simulink model "M2C_IM_CL_V1_NCADMM_Sim"  (R2023a)
settings: Solver=ode4  StartTime=0.0  StopTime=t_sim  FixedStep=tsim  RelTol=1e-3
model workspace (MAT data in the model file):
  global_can_baud_rate = '1000000'
  global_ip_addresses : object (value not decoded)
values from neighbouring files (symbols this model uses):
  A = [1 1 1 0 0 0 ... (first row only)    [M2C_init.m]    (also in MMCC_Sim_Script_BCD_activeset.m = -[1 0 0 1 0 0 1 0 0; 0 1 0 0 1 0 0 1 0; 0 0 1 0 0 1 0 0 1; -; MMCC_Sim_Script_BCD_activeset_LH.m = -[1 0 0 1 0 0 1 0 0; 0 1 0 0 1 0 0 1 0; 0 0 1 0 0 1 0 0 1; -)
  A11 = -(1/tau_sig)*eye(2)    [M2C_init.m]
  A21 = (Lm/tau_r)*eye(2)    [M2C_init.m]
  A_admm = zeros(2*Np, Np)    [M2C_init.m]
  A_cc = [1 0 ... (first row only)    [M2C_init.m]
  b_admm_1 = imax_admm*ones(2*Np,1)    [M2C_init.m]
  b_cc = Vmax_cc*ones(4,1)    [M2C_init.m]
  c_admm = -imax_admm*ones(Np,1)    [M2C_init.m]
  C_obs = [eye(2) zeros(2)]    [M2C_init.m]
  C_sm = 987e-6    (= 0.000987)    [M2C_init.m]
  G_cc = [1 1 ... (first row only)    [M2C_init.m]
  J_imag = [0 -1 ... (first row only)    [M2C_init.m]
  K_obsm = K_obs2'    [M2C_init.m]
  K_obsp = K_obs1'    [M2C_init.m]
  kr = Lm/Lr    (= 0.989061842659)    [M2C_init.m]
  L = 5e-3    (= 0.005)    [M2C_init.m]    (also in MMCC_Sim_Script_BCD_activeset.m = 0.02; MMCC_Sim_Script_BCD_activeset_LH.m = 0.02)
  Lsigmar = 2.6e-3    (= 0.0026)    [M2C_init.m]
  Lsigmas = 2.6e-3    (= 0.0026)    [M2C_init.m]
  N = [1/sqrt(3) 0;-1/(2*sqrt(3)) 1/2;-1/(2*sqrt(3)) -1/2;-1/sqrt(3) 0;1/(2*sqrt(3)) -1/2;1/(2*sqrt(3)) 1/2]    [M2C_init.m]    (also in MMCC_Sim_Script_BCD_activeset.m = null(A,'rational'); MMCC_Sim_Script_BCD_activeset_LH.m = [-0.4430   -0.4780    0.0994    0.0994)
  n = 4    [M2C_init.m]
  p = 2    [M2C_init.m]
  phirN = 1*Vb/ws_nom    [M2C_init.m]
  prmt_ADMM = [n, lambda_z, rho, lambda_e, C_sm, Np, imax_admm]    [M2C_init.m]
  prmt_bkpsi = [ts, Np, lambda_o, imax_admm]    [M2C_init.m]
  prmt_CCMPC = [ts, L, lambda_u, lambda_i, R, e]    [M2C_init.m]
  prmt_OBS = [ts, kr, sigma, Ls, tau_r]    [M2C_init.m]
  R = 0.2    [M2C_init.m]    (also in MMCC_Sim_Script_BCD_activeset.m = 0.001; MMCC_Sim_Script_BCD_activeset_LH.m = 0.001)
  Rr = 1.8    [M2C_init.m]
  Rs = 1.8    [M2C_init.m]
  Rsig = Rs + Rr*kr^2    (= 3.56083799149)    [M2C_init.m]
  SN = PN/FPn    (= 3703.7037037)    [M2C_init.m]
  T = [An ... (first row only)    [M2C_init.m]    (also in MMCC_Sim_Script_BCD_activeset.m = [1   0 ; -1/2  sqrt(3)/2; -1/2  -sqrt(3)/2]; MMCC_Sim_Script_BCD_activeset_LH.m = [1   0 ; -1/2  sqrt(3)/2; -1/2  -sqrt(3)/2])
  t_arranque = t_flux + 5/(dam*wn_flux) + 0.4    [M2C_init.m]
  t_flux = t_maq + 0.1    (= 0.3)    [M2C_init.m]
  t_load = t_arranque    [M2C_init.m]
  Tab0 = (1/3)*[2 -1 -1 ... (first row only)    [M2C_init.m]
  Tabc = [1 0; -.5 sqrt(3)/2; -.5 -sqrt(3)/2]    [M2C_init.m]
  tau_r = Lr/Rr    (= 0.132055555556)    [M2C_init.m]
  TN = PN/(nN*pi/30)    (= 19.7571653493)    [M2C_init.m]
  ts = 1/fs    (= 0.000166666666667)    [M2C_init.m]
  tsim = ts/40    (= 4.16666666667e-06)    [M2C_init.m]
  Vc0 = n*Vc_sm    (= 520)    [M2C_init.m]    (also in MMCC_Sim_Script_BCD_activeset.m = 18000; MMCC_Sim_Script_BCD_activeset_LH.m = 18000)
  Vc_sm = 130    [M2C_init.m]
  Vdc = n*Vc_sm    (= 520)    [M2C_init.m]
undefined symbols (not defined in the file or in its folder): Down, M2C_ADMM_Init_IM_V1, plecs, Up
libraries: spsIGBTDiodeLib x48, spsVoltageMeasurementLib x36, spsSeriesRLCBranchLib x30, spsCurrentMeasurementLib x10, eePwmGenerator x6, rtlab x3, dspstat3 x2, spsControlledVoltageSourceLib x2, spsDCVoltageSourceLib x2, opal_lib x1, dspfdesign x1, spsMeanLib x1
(part 5 of 6)

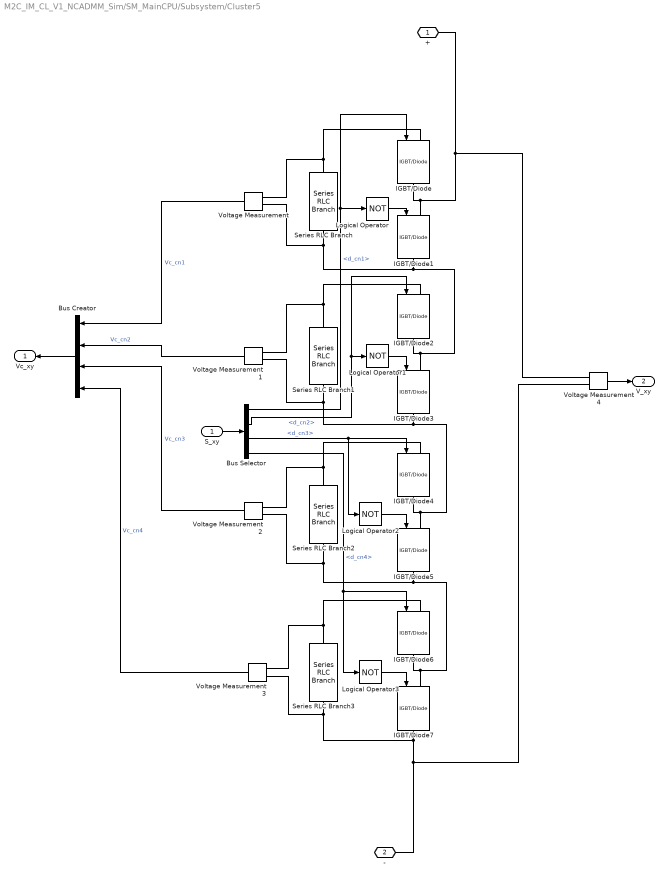
== system M2C_IM_CL_V1_NCADMM_Sim/SM_MainCPU/Subsystem/Cluster5 ==
  S_xy : Inport
  Bus Creator : BusCreator  Inputs=4
  Bus Selector : BusSelector  OutputSignals=d_cn1,d_cn2,d_cn3,d_cn4
  IGBT/Diode{,1..7} (8 alike) : spsIGBTDiodeLib/IGBT//Diode  Ron=1e-5  Rs=1e5  Cs=inf  Measurements=off
  Logical Operator{,1..3} (4 alike) : Logic  Operator=NOT  AllPortsSameDT=off  OutDataTypeStr=boolean
  Series RLC Branch{,1..3} (4 alike) : spsSeriesRLCBranchLib/Series RLC Branch  LConnTagsString=__new0  RConnTagsString=__new0  BranchType=C  Resistance=1  Inductance=1e-3  SetiL0=off  InitialCurrent=0  Capacitance=C_sm  Setx0=on  InitialVoltage=V0c  Measurements=None
  Voltage Measurement{,1..4} (5 alike) : spsVoltageMeasurementLib/Voltage Measurement  PhasorSimulation=off  OutputType=Complex  PSBequivalent=0
  + : PMIOPort  Side=Left
  - : PMIOPort  Port=2  Side=Right
  Vc_xy : Outport
  V_xy : Outport  Port=2
  wires:
  Bus Selector/4 -> IGBT/Diode6/1, Logical Operator3/1  "<d_cn4>"
  Bus Selector/3 -> IGBT/Diode4/1, Logical Operator2/1  "<d_cn3>"
  Bus Selector/2 -> IGBT/Diode2/1, Logical Operator1/1  "<d_cn2>"
  Bus Selector/1 -> Logical Operator/1, IGBT/Diode/1  "<d_cn1>"
  S_xy/1 -> Bus Selector/1
  Logical Operator/1 -> IGBT/Diode1/1
  Logical Operator1/1 -> IGBT/Diode3/1
  Logical Operator2/1 -> IGBT/Diode5/1
  Logical Operator3/1 -> IGBT/Diode7/1
  Bus Creator/1 -> Vc_xy/1
  Voltage Measurement3/1 -> Bus Creator/4  "Vc_cn4"
  Voltage Measurement2/1 -> Bus Creator/3  "Vc_cn3"
  Voltage Measurement1/1 -> Bus Creator/2  "Vc_cn2"
  Voltage Measurement/1 -> Bus Creator/1  "Vc_cn1"
  Voltage Measurement4/1 -> V_xy/1
  connections:
  Voltage Measurement1/LConn1 -- Series RLC Branch1/LConn1 -- IGBT/Diode2/LConn1
  Voltage Measurement2/LConn1 -- Series RLC Branch2/LConn1 -- IGBT/Diode4/LConn1
  Voltage Measurement/LConn2 -- Series RLC Branch/RConn1 -- IGBT/Diode3/LConn1 -- IGBT/Diode2/RConn1 -- IGBT/Diode1/RConn1
  Voltage Measurement1/LConn2 -- Series RLC Branch1/RConn1 -- IGBT/Diode3/RConn1 -- IGBT/Diode4/RConn1 -- IGBT/Diode5/LConn1
  Voltage Measurement/LConn1 -- Series RLC Branch/LConn1 -- IGBT/Diode/LConn1
  Voltage Measurement3/LConn1 -- Series RLC Branch3/LConn1 -- IGBT/Diode6/LConn1
  Voltage Measurement3/LConn2 -- Series RLC Branch3/RConn1 -- IGBT/Diode7/RConn1 -- Voltage Measurement4/LConn1 -- -/RConn1
  Voltage Measurement2/LConn2 -- Series RLC Branch2/RConn1 -- IGBT/Diode5/RConn1 -- IGBT/Diode6/RConn1 -- IGBT/Diode7/LConn1
  IGBT/Diode/RConn1 -- IGBT/Diode1/LConn1 -- +/RConn1 -- Voltage Measurement4/LConn2

== system M2C_IM_CL_V1_NCADMM_Sim/SM_MainCPU/Subsystem/Scope ==
  1 : Inport
  " InputMux " : Subsystem
      mask Display: disp('Mux')
  " S-Function " : S-Function  FunctionName=plecs  SFunctionDeploymentMode=off  EnableBusSupport=off
  wires:
  1/1 -> " InputMux "/1(In1)
  " InputMux "/1(Out) -> " S-Function "/1

== system M2C_IM_CL_V1_NCADMM_Sim/SM_MainCPU/Subsystem/Scope1 ==
  1 : Inport
  " InputMux " : Subsystem
      mask Display: disp('Mux')
  " S-Function " : S-Function  FunctionName=plecs  SFunctionDeploymentMode=off  EnableBusSupport=off
  wires:
  1/1 -> " InputMux "/1(In1)
  " InputMux "/1(Out) -> " S-Function "/1

== system M2C_IM_CL_V1_NCADMM_Sim/SM_MainCPU/Subsystem/Scope2 ==
  1 : Inport
  " InputMux " : Subsystem
      mask Display: disp('Mux')
  " S-Function " : S-Function  FunctionName=plecs  SFunctionDeploymentMode=off  EnableBusSupport=off
  wires:
  1/1 -> " InputMux "/1(In1)
  " InputMux "/1(Out) -> " S-Function "/1

== system M2C_IM_CL_V1_NCADMM_Sim/SM_MainCPU/Subsystem/Scope3 ==
  1 : Inport
  " InputMux " : Subsystem
      mask Display: disp('Mux')
  " S-Function " : S-Function  FunctionName=plecs  SFunctionDeploymentMode=off  EnableBusSupport=off
  wires:
  1/1 -> " InputMux "/1(In1)
  " InputMux "/1(Out) -> " S-Function "/1

== system M2C_IM_CL_V1_NCADMM_Sim/SM_MainCPU/Subsystem/Scope4 ==
  1 : Inport
  " InputMux " : Subsystem
      mask Display: disp('Mux')
  " S-Function " : S-Function  FunctionName=plecs  SFunctionDeploymentMode=off  EnableBusSupport=off
  wires:
  1/1 -> " InputMux "/1(In1)
  " InputMux "/1(Out) -> " S-Function "/1

== system M2C_IM_CL_V1_NCADMM_Sim/SM_MainCPU/Subsystem/Scope5 ==
  1 : Inport
  " InputMux " : Subsystem
      mask Display: disp('Mux')
  " S-Function " : S-Function  FunctionName=plecs  SFunctionDeploymentMode=off  EnableBusSupport=off
  wires:
  1/1 -> " InputMux "/1(In1)
  " InputMux "/1(Out) -> " S-Function "/1

== system M2C_IM_CL_V1_NCADMM_Sim/SM_MainCPU/Subsystem/Scope6 ==
  1 : Inport
  " InputMux " : Subsystem
      mask Display: disp('Mux')
  " S-Function " : S-Function  FunctionName=plecs  SFunctionDeploymentMode=off  EnableBusSupport=off
  wires:
  1/1 -> " InputMux "/1(In1)
  " InputMux "/1(Out) -> " S-Function "/1

== system M2C_IM_CL_V1_NCADMM_Sim/SM_MainCPU/LCB1/Scope/ InputMux  ==
  In1 : Inport
  Convert1 : DataTypeConversion
  Mux : Mux  Inputs=1
  Out : Outport
  wires:
  Convert1/1 -> Mux/1
  In1/1 -> Convert1/1
  Mux/1 -> Out/1

== system M2C_IM_CL_V1_NCADMM_Sim/SM_MainCPU/LCB1/Scope1/ InputMux  ==
  In1 : Inport
  Convert1 : DataTypeConversion
  Mux : Mux  Inputs=1
  Out : Outport
  wires:
  Convert1/1 -> Mux/1
  In1/1 -> Convert1/1
  Mux/1 -> Out/1

== system M2C_IM_CL_V1_NCADMM_Sim/SM_MainCPU/LCB1/Scope2/ InputMux  ==
  In1 : Inport
  Convert1 : DataTypeConversion
  Mux : Mux  Inputs=1
  Out : Outport
  wires:
  Convert1/1 -> Mux/1
  In1/1 -> Convert1/1
  Mux/1 -> Out/1

== system M2C_IM_CL_V1_NCADMM_Sim/SM_MainCPU/LCB1/Scope5/ InputMux  ==
  In1 : Inport
  Convert1 : DataTypeConversion
  Mux : Mux  Inputs=1
  Out : Outport
  wires:
  Convert1/1 -> Mux/1
  In1/1 -> Convert1/1
  Mux/1 -> Out/1

== system M2C_IM_CL_V1_NCADMM_Sim/SM_MainCPU/Subsystem/Cluster/Scope ==
  1 : Inport
  " InputMux " : Subsystem
      mask Display: disp('Mux')
  " S-Function " : S-Function  FunctionName=plecs  SFunctionDeploymentMode=off  EnableBusSupport=off
  wires:
  1/1 -> " InputMux "/1(In1)
  " InputMux "/1(Out) -> " S-Function "/1

== system M2C_IM_CL_V1_NCADMM_Sim/SM_MainCPU/Subsystem/Cluster/Scope1 ==
  1 : Inport
  " InputMux " : Subsystem
      mask Display: disp('Mux')
  " S-Function " : S-Function  FunctionName=plecs  SFunctionDeploymentMode=off  EnableBusSupport=off
  wires:
  1/1 -> " InputMux "/1(In1)
  " InputMux "/1(Out) -> " S-Function "/1

== system M2C_IM_CL_V1_NCADMM_Sim/SM_MainCPU/Subsystem/Cluster/Scope2 ==
  1 : Inport
  " InputMux " : Subsystem
      mask Display: disp('Mux')
  " S-Function " : S-Function  FunctionName=plecs  SFunctionDeploymentMode=off  EnableBusSupport=off
  wires:
  1/1 -> " InputMux "/1(In1)
  " InputMux "/1(Out) -> " S-Function "/1

== system M2C_IM_CL_V1_NCADMM_Sim/SM_MainCPU/Subsystem/Cluster/Scope3 ==
  1 : Inport
  " InputMux " : Subsystem
      mask Display: disp('Mux')
  " S-Function " : S-Function  FunctionName=plecs  SFunctionDeploymentMode=off  EnableBusSupport=off
  wires:
  1/1 -> " InputMux "/1(In1)
  " InputMux "/1(Out) -> " S-Function "/1

== system M2C_IM_CL_V1_NCADMM_Sim/SM_MainCPU/Subsystem/Scope/ InputMux  ==
  In1 : Inport
  Convert1 : DataTypeConversion
  Mux : Mux  Inputs=1
  Out : Outport
  wires:
  Convert1/1 -> Mux/1
  In1/1 -> Convert1/1
  Mux/1 -> Out/1

== system M2C_IM_CL_V1_NCADMM_Sim/SM_MainCPU/Subsystem/Scope1/ InputMux  ==
  In1 : Inport
  Convert1 : DataTypeConversion
  Mux : Mux  Inputs=1
  Out : Outport
  wires:
  Convert1/1 -> Mux/1
  In1/1 -> Convert1/1
  Mux/1 -> Out/1

== system M2C_IM_CL_V1_NCADMM_Sim/SM_MainCPU/Subsystem/Scope2/ InputMux  ==
  In1 : Inport
  Convert1 : DataTypeConversion
  Mux : Mux  Inputs=1
  Out : Outport
  wires:
  Convert1/1 -> Mux/1
  In1/1 -> Convert1/1
  Mux/1 -> Out/1

== system M2C_IM_CL_V1_NCADMM_Sim/SM_MainCPU/Subsystem/Scope3/ InputMux  ==
  In1 : Inport
  Convert1 : DataTypeConversion
  Mux : Mux  Inputs=1
  Out : Outport
  wires:
  Convert1/1 -> Mux/1
  In1/1 -> Convert1/1
  Mux/1 -> Out/1

== system M2C_IM_CL_V1_NCADMM_Sim/SM_MainCPU/Subsystem/Scope4/ InputMux  ==
  In1 : Inport
  Convert1 : DataTypeConversion
  Mux : Mux  Inputs=1
  Out : Outport
  wires:
  Convert1/1 -> Mux/1
  In1/1 -> Convert1/1
  Mux/1 -> Out/1

== system M2C_IM_CL_V1_NCADMM_Sim/SM_MainCPU/Subsystem/Scope5/ InputMux  ==
  In1 : Inport
  Convert1 : DataTypeConversion
  Mux : Mux  Inputs=1
  Out : Outport
  wires:
  Convert1/1 -> Mux/1
  In1/1 -> Convert1/1
  Mux/1 -> Out/1

== system M2C_IM_CL_V1_NCADMM_Sim/SM_MainCPU/Subsystem/Scope6/ InputMux  ==
  In1 : Inport
  Convert1 : DataTypeConversion
  Mux : Mux  Inputs=1
  Out : Outport
  wires:
  Convert1/1 -> Mux/1
  In1/1 -> Convert1/1
  Mux/1 -> Out/1

== system M2C_IM_CL_V1_NCADMM_Sim/SM_MainCPU/Subsystem/Cluster/Scope/ InputMux  ==
  In1 : Inport
  Convert1 : DataTypeConversion
  Mux : Mux  Inputs=1
  Out : Outport
  wires:
  Convert1/1 -> Mux/1
  In1/1 -> Convert1/1
  Mux/1 -> Out/1

== system M2C_IM_CL_V1_NCADMM_Sim/SM_MainCPU/Subsystem/Cluster/Scope1/ InputMux  ==
  In1 : Inport
  Convert1 : DataTypeConversion
  Mux : Mux  Inputs=1
  Out : Outport
  wires:
  Convert1/1 -> Mux/1
  In1/1 -> Convert1/1
  Mux/1 -> Out/1

== system M2C_IM_CL_V1_NCADMM_Sim/SM_MainCPU/Subsystem/Cluster/Scope2/ InputMux  ==
  In1 : Inport
  Convert1 : DataTypeConversion
  Mux : Mux  Inputs=1
  Out : Outport
  wires:
  Convert1/1 -> Mux/1
  In1/1 -> Convert1/1
  Mux/1 -> Out/1

== system M2C_IM_CL_V1_NCADMM_Sim/SM_MainCPU/Subsystem/Cluster/Scope3/ InputMux  ==
  In1 : Inport
  Convert1 : DataTypeConversion
  Mux : Mux  Inputs=1
  Out : Outport
  wires:
  Convert1/1 -> Mux/1
  In1/1 -> Convert1/1
  Mux/1 -> Out/1

== matlab function M2C_IM_CL_V1_NCADMM_Sim/SM_MainCPU/SOFTWARE PROTECTIONS ==
  data: max_vcap input; log output; min_vcap input; Pm input; iarm input; en_user input; en output
function [log, en] = fcn(max_vcap, min_vcap, Pm, iarm, en_user)
% protecciones de software contra sobre voltajes y corrientes. El log
% permite al gui saber si hubo falla o no
% log = 0 en_user = 0
% log = 1 sin fallas
% log = 2 falla de voltage
% log = 3 falla de corriente

persistent en0 log0
if isempty(en0)
    en0 = 1;
    log0 = 1;
end

%% falla de voltaje
if (max_vcap >= 170) && en0 == 1
    en0 = 0;
    log0 = 2; 
end

%% falla de corriente
if (iarm >= 18) && en0 == 1
    en0 = 0;
    log0 = 3; 
end

%% falla de corriente
if (Pm <= -1500) && en0 == 1
    en0 = 0;
    log0 = 4; 
end

en = en_user*en0;
log = log0;

== matlab function M2C_IM_CL_V1_NCADMM_Sim/SM_MainCPU/FAULT ID ==
  settings: sampleTime=ts
  data: EN input; ID_fault output; log input; Vcaps input; Iyx input; Fault_value output; Pm input
function [ID_fault,Fault_value]=    fcn(EN,log, Vcaps, Iyx, Pm)

persistent ID F
if isempty(ID)
    F = 0;
    ID = 0;
end
if EN==0
    if log==0       %User End
        F=0;
        ID=0;
    elseif log==2 && ID == 0  %Falla de voltaje
        [F,ID] = max(Vcaps);
    elseif log==3 && ID == 0  %Falla de corriente
        [F,ID] = max(Iyx);
        F=abs(F);
    elseif log==4 && ID == 0  %Falla de corriente
        F = Pm;
        ID = 4;
    end
end
ID_fault=ID;
Fault_value=F;
end

== matlab function M2C_IM_CL_V1_NCADMM_Sim/SM_MainCPU/dq --> ab ==
  settings: updateMethod=DISCRETE  sampleTime=ts
  data: dq input; ab output; Theta_s input
function ab = fcn(dq, Theta_s)

Tab = [cos(Theta_s) -sin(Theta_s);
      sin(Theta_s) cos(Theta_s)];
ab = Tab*dq;

== matlab function M2C_IM_CL_V1_NCADMM_Sim/SM_MainCPU/Flux Control Proportional Control1 ==
  settings: updateMethod=DISCRETE  sampleTime=ts
  data: in input; id_ref output; prmt_FC parameter; En input
function id_ref = fcn(in, prmt_FC, En)
% 3 inputs
% 1 output
% 5 parameters

psir = in(1);
psir_ref = in(2);

Kpt = prmt_FC(1)/1.5;
imax = prmt_FC(2);
ts = prmt_FC(3);
Lm = prmt_FC(4);

im_r = psir/Lm;
im_rr = psir_ref/Lm;

im_rr = im_rr*(Kpt + 1)/Kpt;

% nct = 1 - ts*0.5*Kit/Kpt;

% error
persistent a 
if isempty(a)
    a = 0;
end

% % antiwindup signal
persistent u
if isempty(u)
    u = 0;
end


%% PI antiwindup
e1 = (im_rr - im_r);


% a = (nct - 1)*u/Kpt + a*nct;
% u = (e1 - a)*Kpt;


% if u >= imax
%     u = imax;
% elseif u <= -imax
%     u = -imax;
% end

u2 = Kpt*e1;

if u2 >= imax
    u2 = imax;
elseif u2 <= -imax
    u2 = -imax;
end

id_ref = En*u2;

== matlab function M2C_IM_CL_V1_NCADMM_Sim/SM_MainCPU/Speed Control Proportional Integral Control1 ==
  settings: updateMethod=DISCRETE  sampleTime=6*ts
  data: in input; iq_ref output; prmt_SC parameter; En input
function iq_ref = fcn(in, prmt_SC, En)
% 3 inputs
% 1 output
% 5 parameters

w = in(1);
w_ref = in(2);

Kpt = prmt_SC(1);
nct = prmt_SC(2);
imax = prmt_SC(3);
% Adc = prmt_SC(4);
ts = prmt_SC(4);

% nct = 1 - ts*0.5*Kit/Kpt;

% error
persistent a 
if isempty(a)
    a = 0;
end

% % antiwindup signal
persistent u
if isempty(u)
    u = 0;
end


%% PI antiwindup
e1 = (w_ref - w);

a = (nct - 1)*u/Kpt + a*nct;
u = (e1 - a)*Kpt;

if u >= imax
    u = imax;
elseif u <= -imax
    u = -imax;
end


iq_ref = En*u;

== matlab function M2C_IM_CL_V1_NCADMM_Sim/SM_MainCPU/MATLAB Function ==
  data: u input; y output
function y = fcn(u)
N=[1/sqrt(3) 0;-1/(2*sqrt(3)) 1/2;-1/(2*sqrt(3)) -1/2;-1/sqrt(3) 0;1/(2*sqrt(3)) -1/2;1/(2*sqrt(3)) 1/2];
y=N*N'*u;

== matlab function M2C_IM_CL_V1_NCADMM_Sim/SM_MainCPU/ADMM Horizonte Np/ADMM Corriente AIO ==
  settings: updateMethod=DISCRETE  sampleTime=ts
  data: i_kopt output; v_oopt output; V_ck input; prmt_ADMM parameter; prmt_bkpsi parameter; A parameter; v_dc_ab input; i_dc_albet input; v_o input; N output; criterio output; w input; c_admm parameter; debug output; En_admm input; lambda_z input; lambda_0 input; A_admm parameter; b_admm_1 parameter; Tabc parameter
function [i_kopt,v_oopt, N, criterio, debug] = ADMM(V_ck, prmt_ADMM, prmt_bkpsi,A,v_dc_ab,i_dc_albet,v_o, w, c_admm,  En_admm, lambda_z, lambda_0, A_admm, b_admm_1, Tabc)
% 6 inputs
% 1 output
% 4 parameters
% 1 Persistent

% v_abc_uvw tensiones de cada fase como vector 5 x 1 orden [p m a b c]
% i_abc_uvw corrientes por rama solo componente de fases como vector 6 x 1 orden [pa pb pc ma mb mc]
% i_z corrientes de rama solo componente circulante (las de referencia)

Ts = prmt_bkpsi(1); Np = prmt_bkpsi(2);
% lambda_o = prmt_bkpsi(3); 
imax = prmt_bkpsi(4);
b_k = zeros(Np+1*0,6);
psi0_k = zeros(Np+1*0,6);
i_xyl = zeros(6,Np+1*0);
v_xyl=zeros(6,Np);

options = mpcActiveSetOptions;
lb = -imax*ones(6,1);
ub = imax*ones(6,1);
iA0 = false(size([ub;-lb]));
i_z0 = zeros(Np+1,6);

v_albet = [v_dc_ab(3) ; v_dc_ab(4)];
i_albet = [i_dc_albet(1) ; i_dc_albet(2)];
idcl = i_dc_albet(3);
vdcl = [v_dc_ab(1) ; v_dc_ab(2)];
persistent v_op
if isempty(v_op)
    v_op=zeros(Np,1);
end


magv_o = v_o(1);
angv_o = v_o(2);
w_m=w;
wo = 150*2*pi;

for l = 0:Np-1+1*0
    wt = (l)*Ts*w_m;
    wot = (l)*Ts*wo;
    iabl = [cos(wt) -sin(wt);
           sin(wt) cos(wt)]*i_albet;
    vabl = [cos(wt) -sin(wt);
           sin(wt) cos(wt)]*[v_albet(1) ; v_albet(2)];

    % Transformación
    vabcl = Tabc*vabl;
    iabcl = Tabc*iabl;
    v_l = [vdcl ; vabcl];
    v_xyl(:,l+1) = A'*v_l;  % [vpa vpb vpc vma vmb vmc] 6 x 1
    ipa = 0.333*idcl - 0.5*iabcl(1);
    ipb = 0.333*idcl - 0.5*iabcl(2);
    ipc = 0.333*idcl - 0.5*iabcl(3);

    ima = -0.333*idcl - 0.5*iabcl(1);
    imb = -0.333*idcl - 0.5*iabcl(2);
    imc = -0.333*idcl - 0.5*iabcl(3);
    
    i_xyl(:,l+1) = [ipa ; ipb ; ipc ; ima ; imb ; imc];

    %v_o = magv_o*(cos(angv_o)*sin(wot) + sin(angv_o)*cos(wot));
    % v_o = magv_o;

   % aux = Ts*(v_xyl + v_o*ones(6,1));

    % vxy = A'*vxypred(k,:);
%     D = diag(v_xyl);
%     Do = diag(v_o*ones(6,1));
%     H = 2*((Ts^2)*(N'*(D + Do)^2)*N + lambda_o*N'*N);
%     u = Ts*(D + Do)*i_xyl(:,l+1);
%     f = 2*Ts*N'*(D + Do)*u;
% 
%     [Z, ~] = mpcActiveSetSolver(H,f,[N;-N],[ub;-lb],zeros(0,length(f)),zeros(0,1),iA0,options);
%     i_z0(l+1,:) = N*Z;

end

n = prmt_ADMM(1); %lambda_z = prmt_ADMM(2);
rho = prmt_ADMM(3); lambda_e = prmt_ADMM(4); 
C = prmt_ADMM(5); Np = prmt_ADMM(6); imax_admm = prmt_ADMM(7);


% if abs(w) >= 20
%     lambda_z = lambda_z*500;
% end

lambdas =  zeros(Np,1);
lambdas(1) = lambda_z;


if Np > 1
    for j = 2:Np
    lambdas(j) = lambda_z;
    end
end
R = diag(lambdas);

persistent i_k0

if isempty(i_k0)
    i_k0 = zeros(6,Np);
end


En = 0.5*C.*V_ck;
En_1 = En;

En_ref = mean(En_1);

Aeq = zeros(0,Np);
beq = zeros(0,1);

opt = mpcActiveSetOptions;


crit = 1;
N = 0;

lambda_d = 0*ones(5*Np,1);

Ak = zeros(5*Np,Np,6);

for j = 1:6
    for l = 0:Np-1
        Ak(5*l+1:5*l+5,l+1,j) = A(:,j);
    end
end

while crit > 10e-3
    N = N + 1;
    for l = 0:Np-1+1*0 %Updated Circulating Current Matrices
        aux = Ts*(v_xyl(:,l+1) + v_op(l+1)*ones(6,1));
        b_k(l+1,:) = aux';
        psi0_k(l+1,:) = (aux.*i_xyl(:,l+1))';
    end
    for j = 1:6 %Circulating Current Subproblems
        % Ak = zeros(5*Np,Np);
        B = zeros(Np,Np);
        C = zeros(Np,1);
%         b_admm = zeros(2*Np,1);
        %j  % Rama
        switch j
            case 1
                for l = 0:Np-1
                    % Ak(5*l+1:5*l+5,l+1) = A(:,j);
                    B(l+1:Np,l+1) = b_k(l+1+1*0,j)*ones(Np-l,1);
                    C(l+1) = i_k0(2,l+1) + i_k0(3,l+1) + i_k0(4,l+1);
%                     b_admm(2*l+1) = imax_admm - i_xyl(j,l+1);
%                     b_admm(2*l+2) = imax_admm + i_xyl(j,l+1);
                end

                PSI0 = tril(ones(Np,Np))*psi0_k(1+1*0:end,j);

                H = 2*(B'*lambda_e*eye(Np)*B + (rho)*eye(Np) + R);
                f = 2*(B'*lambda_e*eye(Np)*(ones(Np,1)*En_1(j,1) + PSI0 - ones(Np,1)*En_ref)) - (lambda_d'*Ak(:,:,j))' + rho*C;
                [Z, ~] = mpcActiveSetSolver(H,f,A_admm,b_admm_1,Aeq,beq,false(size(b_admm_1)),opt);
%                 x_uc = -(H^-1)*f;
%                 [Z, ~] = BoxCQP_Nitmax(length(i_k0(j,:)), H, f, c_admm, b_admm, x_uc, 100);
%                 Z = MPCActSolver(H, f, imax, imax, x_uc);
                i_k0(j,:) = Z;

                
            case 2
                for l = 0:Np-1
                    % Ak(5*l+1:5*l+5,l+1) = A(:,j);
                    B(l+1:Np,l+1) = b_k(l+1+1*0,j)*ones(Np-l,1);
                    C(l+1) = i_k0(1,l+1) + i_k0(3,l+1) + i_k0(5,l+1);
%                     b_admm(2*l+1) = imax_admm - i_xyl(j,l+1);
%                     b_admm(2*l+2) = imax_admm + i_xyl(j,l+1);
                end

                PSI0 = tril(ones(Np,Np))*psi0_k(1+1*0:end,j);

                H = 2*(B'*lambda_e*eye(Np)*B + (rho)*eye(Np) + R);
                f = 2*(B'*lambda_e*eye(Np)*(ones(Np,1)*En_1(j,1) + PSI0 - ones(Np,1)*En_ref)) - (lambda_d'*Ak(:,:,j))' + rho*C;
                [Z, ~] = mpcActiveSetSolver(H,f,A_admm,b_admm_1,Aeq,beq,false(size(b_admm_1)),opt);
%                 x_uc = -(H^-1)*f;
%                 [Z, ~] = BoxCQP_Nitmax(length(i_k0(j,:)), H, f, c_admm, b_admm, x_uc, 100);
%                 Z = MPCActSolver(H, f, imax, imax, x_uc);
                % Z = quadprog(H,f,[],[],[],[],lb,ub,i_k0(j,:),options);
                i_k0(j,:) = Z;

            case 3
                for l = 0:Np-1
                    % Ak(5*l+1:5*l+5,l+1) = A(:,j);
                    B(l+1:Np,l+1) = b_k(l+1+1*0,j)*ones(Np-l,1);
                    C(l+1) = i_k0(1,l+1) + i_k0(2,l+1) + i_k0(6,l+1);
%                     b_admm(2*l+1) = imax_admm - i_xyl(j,l+1);
%                     b_admm(2*l+2) = imax_admm + i_xyl(j,l+1);
                end

                PSI0 = tril(ones(Np,Np))*psi0_k(1+1*0:end,j);

                H = 2*(B'*lambda_e*eye(Np)*B + (rho)*eye(Np) + R);
                f = 2*(B'*lambda_e*eye(Np)*(ones(Np,1)*En_1(j,1) + PSI0 - ones(Np,1)*En_ref)) - (lambda_d'*Ak(:,:,j))' + rho*C;
                [Z, ~] = mpcActiveSetSolver(H,f,A_admm,b_admm_1,Aeq,beq,false(size(b_admm_1)),opt);
%                 x_uc = -(H^-1)*f;
%                 [Z, ~] = BoxCQP_Nitmax(length(i_k0(j,:)), H, f, c_admm, b_admm, x_uc, 100);
%                 Z = MPCActSolver(H, f, imax, imax, x_uc);
                i_k0(j,:) = Z;
                
            case 4
                for l = 0:Np-1
                    % Ak(5*l+1:5*l+5,l+1) = A(:,j);
                    B(l+1:Np,l+1) = b_k(l+1+1*0,j)*ones(Np-l,1);
                    C(l+1) = i_k0(1,l+1) + i_k0(5,l+1) + i_k0(6,l+1);
%                     b_admm(2*l+1) = imax_admm - i_xyl(j,l+1);
%                     b_admm(2*l+2) = imax_admm + i_xyl(j,l+1);
                end

                PSI0 = tril(ones(Np,Np))*psi0_k(1+1*0:end,j);

                H = 2*(B'*lambda_e*eye(Np)*B + (rho)*eye(Np) + R);
                f = 2*(B'*lambda_e*eye(Np)*(ones(Np,1)*En_1(j,1) + PSI0 - ones(Np,1)*En_ref)) - (lambda_d'*Ak(:,:,j))' + rho*C;
                [Z, ~] = mpcActiveSetSolver(H,f,A_admm,b_admm_1,Aeq,beq,false(size(b_admm_1)),opt);
%                 x_uc = -(H^-1)*f;
%                 [Z, ~] = BoxCQP_Nitmax(length(i_k0(j,:)), H, f, c_admm, b_admm, x_uc, 100);
%                 Z = MPCActSolver(H, f, imax, imax, x_uc);
                i_k0(j,:) = Z;
                
            case 5
                for l = 0:Np-1
                    % Ak(5*l+1:5*l+5,l+1) = A(:,j);
                    B(l+1:Np,l+1) = b_k(l+1+1*0,j)*ones(Np-l,1);
                    C(l+1) = i_k0(2,l+1) + i_k0(4,l+1) + i_k0(6,l+1);
%                     b_admm(2*l+1) = imax_admm - i_xyl(j,l+1);
%                     b_admm(2*l+2) = imax_admm + i_xyl(j,l+1);
                end

                PSI0 = tril(ones(Np,Np))*psi0_k(1+1*0:end,j);

                H = 2*(B'*lambda_e*eye(Np)*B + (rho)*eye(Np) + R);
                f = 2*(B'*lambda_e*eye(Np)*(ones(Np,1)*En_1(j,1) + PSI0 - ones(Np,1)*En_ref)) - (lambda_d'*Ak(:,:,j))' + rho*C;
                [Z, ~] = mpcActiveSetSolver(H,f,A_admm,b_admm_1,Aeq,beq,false(size(b_admm_1)),opt);
%                 x_uc = -(H^-1)*f;
%                 [Z, ~] = BoxCQP_Nitmax(length(i_k0(j,:)), H, f, c_admm, b_admm, x_uc, 100);
%                 Z = MPCActSolver(H, f, imax, imax, x_uc);
                i_k0(j,:) = Z;
                
            case 6
                for l = 0:Np-1
                    % Ak(5*l+1:5*l+5,l+1) = A(:,j);
                    B(l+1:Np,l+1) = b_k(l+1+1*0,j)*ones(Np-l,1);
                    C(l+1) = i_k0(3,l+1) + i_k0(4,l+1) + i_k0(5,l+1);
%                     b_admm(2*l+1) = imax_admm - i_xyl(j,l+1);
%                     b_admm(2*l+2) = imax_admm + i_xyl(j,l+1);
                end

                PSI0 = tril(ones(Np,Np))*psi0_k(1+1*0:end,j);

                H = 2*(B'*lambda_e*eye(Np)*B + (rho)*eye(Np) + R);
                f = 2*(B'*lambda_e*eye(Np)*(ones(Np,1)*En_1(j,1) + PSI0 - ones(Np,1)*En_ref)) - (lambda_d'*Ak(:,:,j))' + rho*C;
                [Z, ~] = mpcActiveSetSolver(H,f,A_admm,b_admm_1,Aeq,beq,false(size(b_admm_1)),opt);
%                 x_uc = -(H^-1)*f;
%                 [Z, ~] = BoxCQP_Nitmax(length(i_k0(j,:)), H, f, c_admm, b_admm, x_uc, 100);
%                 Z = MPCActSolver(H, f, imax, imax, x_uc);
                i_k0(j,:) = Z;

        end
    end

    B0 = zeros(6*Np,Np); %CMV subproblem matrices
    d0 = zeros(6*Np,1);
    for l=0:Np-1
        B0((6*l+1):6*Np,l+1)=repmat(Ts*(i_xyl(:,l+1)+i_k0(:,l+1)),Np-l,1);
        if l==0
            d0((6*l+1):(6*l+6))=Ts*v_xyl(:,l+1).*(i_xyl(:,l+1)+i_k0(:,l+1));
        else
            d0((6*l+1):(6*l+6))=Ts*v_xyl(:,l+1).*(i_xyl(:,l+1)+i_k0(:,l+1))+d0((6*(l-1)+1):(6*(l-1)+6));
        end
    end
    
    H=2*(B0'*B0+eye(Np)*lambda_0);
    f=2*(B0'*(repmat(En_1,Np,1)-En_ref*ones(6*Np,1)+d0));
    v0g=abs(1-abs(w_m/(100*pi)));
    if v0g>1
        v0g=1;
    elseif v0g<0
        v0g=0;
    end
    lb=-260*0.8*(1-abs(0/(100*pi)))*ones(Np,1);
    ub=260*0.8*(1-abs(0/(100*pi)))*ones(Np,1);    
    [Z, ~] = mpcActiveSetSolver(H,f,[eye(Np);-eye(Np)],[ub;-lb],zeros(0,length(f)),zeros(0,1),false(size([ones(Np,1);ones(Np,1)])),opt);
    v_op=Z;
    sum_nk = zeros(5*Np,1);
    % Crear suma de corrientes circulantes
    for l = 1:6
        sum_nk = sum_nk + Ak(:,:,l)*(i_k0(l,:))';
    end
    lambda_d = lambda_d - rho*sum_nk;
    crit = norm(sum_nk);
end


criterio = crit;
i_kopt = En_admm*i_k0(:,1);
v_oopt=En_admm*v_op(1);
debug = lambda_z;

== matlab function M2C_IM_CL_V1_NCADMM_Sim/SM_MainCPU/MPC-Deadbeat Current Control2 ==
  settings: updateMethod=DISCRETE  sampleTime=ts
  data: ixyr input; Y output; ixy input; vx input; vy input; diz input; izr input; iz input; ixr input; dixr input; iyr input; diyr input; von input; vcxy input; lambda input; lambdae input; deb output
function [Y, deb] = fcn(ixyr,ixy,vx,vy,diz,izr,iz,ixr,dixr,iyr,diyr,von,vcxy,lambda,lambdae)
% transformada doble alpha beta 0
iarr=ixyr(1); ibrr=ixyr(2); icrr=ixyr(3);
iasr=ixyr(4); ibsr=ixyr(5); icsr=ixyr(6);
%iatr=ixyr(7); ibtr=ixyr(8); ictr=ixyr(9);
ixyr1=[iarr;ibrr;icrr;iasr;ibsr;icsr];
ixy1=[ixy(1);ixy(2);ixy(3);ixy(4);ixy(5);ixy(6)];
ixr1=[ixr(1);ixr(2);ixr(3);ixr(4);ixr(5);ixr(6)];
dixr1=[dixr(1);dixr(2);dixr(3);dixr(4);dixr(5);dixr(6)];
iyr1=[iyr(1);iyr(2);iyr(3);iyr(4);iyr(5);iyr(6)];
diyr1=[diyr(1);diyr(2);diyr(3);diyr(4);diyr(5);diyr(6)];
V0=sqrt(195608196);
va=vx(1); vb=vx(2); vc=vx(3);
vr=vy(1); vs=vy(2); %vt=vy(3);
vz=zeros(6,1);
%A=[1 1 1 0 0 0 0 0 0; 0 0 0 1 1 1 0 0 0; 0 0 0 0 0 0 1 1 1; -1 0 0 -1 0 0 -1 0 0; 0 -1 0 0 -1 0 0 -1 0; 0 0 -1 0 0 -1 0 0 -1];
A=[1 1 1 0 0 0;0 0 0 1 1 1; -1 0 0 -1 0 0;0 -1 0 0 -1 0; 0 0 -1 0 0 -1];
N=[1/sqrt(3) 0;-1/(2*sqrt(3)) 1/2;-1/(2*sqrt(3)) -1/2;-1/sqrt(3) 0;1/(2*sqrt(3)) -1/2;1/(2*sqrt(3)) 1/2];
T=(2/3)*[1 -1/2 -1/2;0 sqrt(3)/2 -sqrt(3)/2];
P=[ 1   0 ; -1/2  sqrt(3)/2; -1/2  -sqrt(3)/2];
ts=1/6000;
L=5e-3; %Arm inductance
R=0.2;			%Arm resistance


vxy=A'*[vr;vs;va;vb;vc];
vyy=A'*[vr;vs;0;0;0];
vxx=A'*[0;0;va;vb;vc];

vxr=vxx-L*dixr1-R*ixr1;
vyr=vyy-L*diyr1-R*iyr1;
vxyr=vxr+vyr-L*diz-R*izr;
%vxyr=vxr+vyr+von*ones(6,1);
%vxyr=vxr+vyr-R*ixyrz-L*dixyrz+von*ones(6,1);

vdb=vxy-(ixyr-ixy)*L/ts;
vis=-(ixyr-ixy)*L/ts;

%    vxyr=vxr+vyr-R*ixyrz-L*dixyrz;
%else
%    vxyr=vxr+vyr;
%end
Q=vxyr;
Q(1:3)=max(Q(1:3),0);
Q(4:6)=min(Q(4:6),0);
%lambda=2.5e-4;
%lambda=3.46e-4; %ts 1e-5
%if t>0.75
%    pl=diag([5 1 1 1 5 1 1 1 5 ]);
%else
pl=eye(6);


%f=2*(-(ts/L)*((1-R*ts/L)*ixy+(ts/L)*vxy+(ts/L)*von*ones(6,1)-ixyr)-lambda*pl*vxyr);

%end
H=2*((ts^2)/(L^2)*eye(6)+lambda*pl);
%vxy=vxx+vxy;
%ixy=(ts/L)*vs0-(ts/L)*vxy+(1-R*ts/L)*ixy;
f=2*(-(ts/L)*((1-R*ts/L)*ixy+(ts/L)*vxy+(ts/L)*von*ones(6,1)-ixyr)-lambda*pl*vxyr);

vunc=H\(-f);
%f=2*((ts/L)*((1-R*ts/L)*ixy+(ts/L)*vxy-(ts/L)*von*ones(6,1)-ixyr)-lambda*pl*vs0*0.2-lambda*pl*vxyr*0.8);
x0 = [0 0 0 0 0 0];
options = mpcActiveSetOptions;
options.MaxIterations = 100;
options.ConstraintTolerance = 1.0e-4;


lb=-vcxy+von*ones(6,1);
lb(1:3)=zeros(3,1)+von*ones(3,1);
ub=vcxy+von*ones(6,1);
ub(4:6)=zeros(3,1)+von*ones(3,1);






iA0=false(size([ub;-lb]));
% %x = quadprog(H,f,A,b,Aeq,beq,lb,ub,x0,options)
% %mpcActiveSetSolver(H,f,A,b,Aeq,beq,iA0,options)
% [Z,exitflag]=mpcActiveSetSolver(H,f,[eye(6);-eye(6)],[ub;-lb],zeros(0,length(f)),zeros(0,1),iA0,options);
% Y=Z-von*ones(6,1);
% f=2*((ts/L)*((1-R*ts/L)*ixy-(ts/L)*vxy-ixyr)-lambda*pl*vxyr);
%f=2*((ts/L)*((1-R*ts/L)*ixy+(ts/L)*vxy-(ts/L)*von*ones(6,1)-ixyr)-lambda*pl*vs0*0.2-lambda*pl*vxyr*0.8);
% x0 = [0 0 0 0 0 0];
% options = mpcActiveSetOptions;
% options.MaxIterations = 100;
% options.ConstraintTolerance = 1.0e-4;
% lb=-vcxy+von*ones(6,1);
% lb(4:6)=zeros(3,1)+von*ones(3,1);
% ub=vcxy+von*ones(6,1);
% ub(1:3)=zeros(3,1)+von*ones(3,1);
% iA0=false(size([ub;-lb]));
%x = quadprog(H,f,A,b,Aeq,beq,lb,ub,x0,options)
%mpcActiveSetSolver(H,f,A,b,Aeq,beq,iA0,options)
[Z,exitflag]=mpcActiveSetSolver(H,f,[eye(6);-eye(6)],[ub;-lb],zeros(0,length(f)),zeros(0,1),iA0,options);
Y=Z-von*ones(6,1);


H=2*((ts^2)/(L^2)*eye(2)+lambdae*eye(2));
f=-2*((ts/L)*((1-R*ts/L)*iz-izr)'*N)';
lb=-(vcxy-Y);
lb(1:3)=zeros(3,1)-Y(1:3);
ub=vcxy-Y;
ub(4:6)=zeros(3,1)-Y(4:6);
options = mpcActiveSetOptions;
options.MaxIterations = 100;
options.ConstraintTolerance = 1.0e-4;
iA0=false(size([ub;-lb]));
[Ve,exitflag]=mpcActiveSetSolver(H,f,[N;-N],[ub;-lb],zeros(0,length(f)),zeros(0,1),iA0,options);
Y=Y+N*Ve;
%Y=Z;
Y(1:3)=max(Y(1:3),0);
Y(4:6)=min(Y(4:6),0);
if vcxy(1)>0
    Ym=Y./vcxy;
else
    Ym=Y./V0;
end
vonMax=min(Z+[vcxy(1:3);zeros(3,1)]);
vonMin=max(Z-[zeros(3,1);vcxy(4:6)]);
%var=(iar-iarr)/(ts/L)+va-vr-R*iar;
%vbr=(ibr-ibrr)/(ts/L)+vb-vr-R*ibr;
%vcr=(icr-icrr)/(ts/L)+vc-vr-R*icr;
%vas=(ias-iasr)/(ts/L)+va-vs-R*ias;
%vbs=(ibs-ibsr)/(ts/L)+vb-vs-R*ibs;
%vcs=(ics-icsr)/(ts/L)+vc-vs-R*ics;
%vat=(iat-iatr)/(ts/L)+va-vt-R*iat;
%vbt=(ibt-ibtr)/(ts/L)+vb-vt-R*ibt;
%vct=(ict-ictr)/(ts/L)+vc-vt-R*ict;
deb = Z;

== matlab function M2C_IM_CL_V1_NCADMM_Sim/SM_MainCPU/I_xy ---> i_x i_y i_xy1 ==
  data: i_xy_measure input; i_x output; i_y output; i_xy output; A parameter
function [i_x,i_y, i_xy] = fcn(i_xy_measure, A)

i_ap = i_xy_measure(1); i_bp = i_xy_measure(2); i_cp = i_xy_measure(3);
i_an = i_xy_measure(4); i_bn = i_xy_measure(5); i_cn = i_xy_measure(6);

i_xy = [-i_ap; -i_bp; -i_cp; -i_an; -i_bn; -i_cn];

i = A*i_xy;

i_x = i(3:5);
i_y = i(1);

== matlab function M2C_IM_CL_V1_NCADMM_Sim/SM_MainCPU/P ==
  settings: updateMethod=DISCRETE  sampleTime=ts
  data: in input; out output
function out = fcn(in)
% 6 inputs
% 2 outputs
% 1 parameter

ia = in(1); ib = in(2);
va = in(3); vb = in(4);

out=zeros(1,1);

Pff=(3/2)*(ia*va + ib*vb);
% Qff=(3/2)*(-vab(1)*iab(2)+vab(2)*iab(1));

out(1)=Pff;

== matlab function M2C_IM_CL_V1_NCADMM_Sim/SM_MainCPU/Torque ==
  settings: updateMethod=DISCRETE  sampleTime=ts
  data: in input; out output; kT parameter
function out = fcn(in, kT)
% 6 inputs
% 2 outputs
% 1 parameter

id = in(1); iq = in(2);
psi = in(3);

out = zeros(1,1);

T = kT*psi*iq;
% Qff=(3/2)*(-vab(1)*iab(2)+vab(2)*iab(1));

out(1) = T;

== matlab function M2C_IM_CL_V1_NCADMM_Sim/SM_MainCPU/LCB1/Greedy ==
  settings: updateMethod=DISCRETE  sampleTime=ts
  data: Vc_xy input; i_xy input; m_xy output; prmt_LCB parameter; Vcr_xy input; EN input; Op_all input; EN_TEB input
function m_xy  = fcn(Vc_xy, i_xy, prmt_LCB, Vcr_xy, EN, Op_all, EN_TEB)

%% Local Balance P controller
n = prmt_LCB(1) ; Vc_prom = prmt_LCB(2); Kc = prmt_LCB(3);

m_xyh = zeros(4,2);
% m_xyl = zeros(4,1);

Vc1 = Vc_xy(1) ; Vc2 = Vc_xy(2); Vc3 = Vc_xy(3); Vc4 = Vc_xy(4);

% d1 = (Vc_prom - Vc1);
% d2 = (Vc_prom - Vc2);
% d3 = (Vc_prom - Vc3);
% d4 = (Vc_prom - Vc4);

d = [Vc1 1; Vc2 2; Vc3 3; Vc4 4];
st_two_w = zeros(2,2);
st_two_l = zeros(2,2);

st_three = zeros(2,2);

% Stage 1 
if Vc1 > Vc2
    st_two_w(1,:) = d(1,:);
    st_two_l(1,:) = d(2,:);
else
    st_two_w(1,:) = d(2,:);
    st_two_l(1,:) = d(1,:);
end
if Vc3 > Vc4
    st_two_w(2,:) = d(3,:);
    st_two_l(2,:) = d(4,:);
else
    st_two_w(2,:) = d(4,:);
    st_two_l(2,:) = d(3,:);
end

% Stage 2
if st_two_w(1,1) > st_two_w(2,1)
    m_xyh(1,:) = st_two_w(1,:);
    st_three(1,:) = st_two_w(2,:);
else
    m_xyh(1,:) = st_two_w(2,:);
    st_three(1,:) = st_two_w(1,:);
end
if st_two_l(1,1) < st_two_l(2,1)
    m_xyh(4,:) = st_two_l(1,:);
    st_three(2,:) = st_two_l(2,:);
else
    m_xyh(4,:) = st_two_l(2,:);
    st_three(2,:) = st_two_l(1,:);
end

%Stage 3
if st_three(1,1) > st_three(2,1)
    m_xyh(2,:) = st_three(1,:);
    m_xyh(3,:) = st_three(2,:);
else
    m_xyh(2,:) = st_three(2,:);
    m_xyh(3,:) = st_three(1,:);
end

if sign(i_xy) > 0
    m_xyh = flip(m_xyh);
end

u_xy = m_xyh(:,1); % Orden de tensiones
n_xy = m_xyh(:,2); % Submodulo al que pertenecen

m_xy = zeros(4,1);
u_sigma = 0;

for i = 1:4
    l = n_xy(i);
    if u_sigma + u_xy(i) <= Vcr_xy
        m_xy(l) = 1;
        u_sigma = u_sigma + u_xy(i);
    else
        m_xy(l) = (Vcr_xy - u_sigma)/u_xy(i);
        if m_xy(l) < 0
            m_xy(l) = 0;
        end
%         if m_xy(l) > 1
%             m_xy(l) = 1;
%         end
        break
    end
end

% m_xy = EN*m_xy;


if Op_all == 1 && EN_TEB == 0
    m_xy = ones(4,1);
else
    m_xy = EN*m_xy;
end






% % Sort h
% for i = 1:4
%     for j = 1:4
%     if i ~= j
%         if d(i) > d(j)
%             m_xyh(i) = m_xyh(i) + 1;
%         end
%     end
%     end
% end
% 
% % Sort l
% for i = 1:4
%     for j = 1:4
%     if i ~= j
%         if d(i) < d(j)
%             m_xyl(i) = m_xyl(i) + 1;
%         end
%     end
%     end
% end
% 
% if sign(i_xy) >= 0
%     m_xy = m_xyh;
% else
%     m_xy = m_xyl;
% end



% for i = 1:4
%     m_xy(i) = Vcrp(i) + d(i);
% end

== matlab function M2C_IM_CL_V1_NCADMM_Sim/SM_MainCPU/Input Current Control Proportional Integral Control ==
  settings: updateMethod=DISCRETE  sampleTime=ts
  data: in input; v_sPref output; prmt_ICC parameter; deb output
function [v_sPref,deb] = fcn(in, prmt_ICC)
% 3 inputs
% 1 output
% 5 parameters

i_P = in(1);
i_Pref = in(2);


Kct = prmt_ICC(1);
nct = prmt_ICC(2);
vmax = prmt_ICC(3);

Adc = in(3);
En = in(4);


% error
persistent a 
if isempty(a)
    a = 0;
end

% % antiwindup signal
persistent u
if isempty(u)
    u = 0;
end


%% PI antiwindup
e1 = (i_Pref - i_P);

a = (nct - 1)*u/Kct + a*nct;
u = (e1 - a)*Kct;

if u >= vmax
    u = vmax;
elseif u <= -vmax
    u = -vmax;
end

deb = u;
v_sPref = En*(u + 1.5*Adc);

== matlab function M2C_IM_CL_V1_NCADMM_Sim/SM_MainCPU/LCB1/Greedy1 ==
  settings: updateMethod=DISCRETE  sampleTime=ts
  data: Vc_xy input; i_xy input; m_xy output; prmt_LCB parameter; Vcr_xy input; EN input; Op_all input; EN_TEB input
function m_xy  = fcn(Vc_xy, i_xy, prmt_LCB, Vcr_xy, EN, Op_all, EN_TEB)

%% Local Balance P controller
n = prmt_LCB(1) ; Vc_prom = prmt_LCB(2); Kc = prmt_LCB(3);

m_xyh = zeros(4,2);
% m_xyl = zeros(4,1);

Vc1 = Vc_xy(1) ; Vc2 = Vc_xy(2); Vc3 = Vc_xy(3); Vc4 = Vc_xy(4);

% d1 = (Vc_prom - Vc1);
% d2 = (Vc_prom - Vc2);
% d3 = (Vc_prom - Vc3);
% d4 = (Vc_prom - Vc4);

d = [Vc1 1; Vc2 2; Vc3 3; Vc4 4];
st_two_w = zeros(2,2);
st_two_l = zeros(2,2);

st_three = zeros(2,2);

% Stage 1 
if Vc1 > Vc2
    st_two_w(1,:) = d(1,:);
    st_two_l(1,:) = d(2,:);
else
    st_two_w(1,:) = d(2,:);
    st_two_l(1,:) = d(1,:);
end
if Vc3 > Vc4
    st_two_w(2,:) = d(3,:);
    st_two_l(2,:) = d(4,:);
else
    st_two_w(2,:) = d(4,:);
    st_two_l(2,:) = d(3,:);
end

% Stage 2
if st_two_w(1,1) > st_two_w(2,1)
    m_xyh(1,:) = st_two_w(1,:);
    st_three(1,:) = st_two_w(2,:);
else
    m_xyh(1,:) = st_two_w(2,:);
    st_three(1,:) = st_two_w(1,:);
end
if st_two_l(1,1) < st_two_l(2,1)
    m_xyh(4,:) = st_two_l(1,:);
    st_three(2,:) = st_two_l(2,:);
else
    m_xyh(4,:) = st_two_l(2,:);
    st_three(2,:) = st_two_l(1,:);
end

%Stage 3
if st_three(1,1) > st_three(2,1)
    m_xyh(2,:) = st_three(1,:);
    m_xyh(3,:) = st_three(2,:);
else
    m_xyh(2,:) = st_three(2,:);
    m_xyh(3,:) = st_three(1,:);
end

if sign(i_xy) > 0
    m_xyh = flip(m_xyh);
end

u_xy = m_xyh(:,1); % Orden de tensiones
n_xy = m_xyh(:,2); % Submodulo al que pertenecen

m_xy = zeros(4,1);
u_sigma = 0;

for i = 1:4
    l = n_xy(i);
    if u_sigma + u_xy(i) <= Vcr_xy
        m_xy(l) = 1;
        u_sigma = u_sigma + u_xy(i);
    else
        m_xy(l) = (Vcr_xy - u_sigma)/u_xy(i);
        if m_xy(l) < 0
            m_xy(l) = 0;
        end
%         if m_xy(l) > 1
%             m_xy(l) = 1;
%         end
        break
    end
end

% m_xy = EN*m_xy;


if Op_all == 1 && EN_TEB == 0
    m_xy = ones(4,1);
else
    m_xy = EN*m_xy;
end






% % Sort h
% for i = 1:4
%     for j = 1:4
%     if i ~= j
%         if d(i) > d(j)
%             m_xyh(i) = m_xyh(i) + 1;
%         end
%     end
%     end
% end
% 
% % Sort l
% for i = 1:4
%     for j = 1:4
%     if i ~= j
%         if d(i) < d(j)
%             m_xyl(i) = m_xyl(i) + 1;
%         end
%     end
%     end
% end
% 
% if sign(i_xy) >= 0
%     m_xy = m_xyh;
% else
%     m_xy = m_xyl;
% end



% for i = 1:4
%     m_xy(i) = Vcrp(i) + d(i);
% end

== matlab function M2C_IM_CL_V1_NCADMM_Sim/SM_MainCPU/n_ref1 ==
  settings: updateMethod=DISCRETE  sampleTime=ts
  data: EN_SC input; n_ref input; time input; n output; Save output
function [n,Save] = fcn(EN_SC, n_ref, time)


persistent t0 
if isempty(t0)
    t0 = 0;
end

persistent x 
if isempty(x)
    x = 0;
end

n = 0;
Save = 0;

if EN_SC == 1 && x == 0
    t0 = time;
    x = 1;
end

if x == 1 && EN_SC == 1
    dt = time - t0;
    if dt <= 11
        Save = 1;
    else
        Save = 0;
    end
    if dt >= 2
        n = EN_SC*n_ref;
    end
    if dt >= 9
        n = -EN_SC*0;
    end
end

== matlab function M2C_IM_CL_V1_NCADMM_Sim/SM_MainCPU/Circulating Current Control MPC ==
  settings: updateMethod=DISCRETE  sampleTime=ts
  data: prmt_CCMPC parameter; ialbet_deltar input size=2; valbet_delta output size=2; ialbet_delta input size=2; G_cc parameter; v_refs input size=4; deb output; Vc_xy input size=6; En input; lambda input; A_cc parameter; b_cc parameter
function [valbet_delta, deb] = fcn(prmt_CCMPC, ialbet_deltar, ialbet_delta, G_cc, v_refs, Vc_xy, En, lambda, A_cc, b_cc)
%MPC Control de corriente

Ts = prmt_CCMPC(1); L = prmt_CCMPC(2);
% lambda = prmt_CCMPC(3); 
lambda_i = prmt_CCMPC(4);
R = prmt_CCMPC(5); e = prmt_CCMPC(6);

persistent ialbet_delr
if isempty(ialbet_delr)
    ialbet_delr = zeros(2,1);
end

% persistent valbet
% if isempty(valbet)
%     valbet = zeros(2,1);
% end

% persistent v_opt
% if isempty(v_opt)
%     v_opt = zeros(2,1);
% end

% Orden de vectores ----> [xaldelta xbetdelta]'

dir = (ialbet_deltar - ialbet_delr)/Ts;

valbet_ref = -L*dir - R*ialbet_deltar;

ex = e^(-R*Ts/L);
G = (1/R)*(ex - 1)*eye(2);
F = ex*eye(2);

% ialbet_delta_1 = F*ialbet_delta + G*valbet;

aux = F*ialbet_delta - ialbet_deltar;

H = 2*(G'*lambda_i*eye(2)*G + lambda*eye(2));

% [L,p] = chol(H,'lower');
% Linv = linsolve(L,eye(size(L)),struct('LT',true));

f = 2*(G'*aux - valbet_ref*lambda*1);
n = length(f);
Aeq = zeros(0,n);
beq = zeros(0,1);


% [Z, ~] = mpcActiveSetSolver(H,f,A_cc,b_cc,Aeq,beq,false(size(b_cc)),opt)
% Z = -(H^-1)*f;

v_sP = v_refs(1); v_salp = v_refs(2); 
v_sbet = v_refs(3); v_s0 = v_refs(4);


v_1 = -0.3333*v_s0 - 0.3333*v_sP + 0.5*v_salp;
v_2 = -0.3333*v_s0 - 0.3333*v_sP - 0.25*v_salp + sqrt(3)*0.25*v_sbet;
v_3 = -0.3333*v_s0 - 0.3333*v_sP - 0.25*v_salp - sqrt(3)*0.25*v_sbet;
v_4 = 0.3333*v_s0 - 0.3333*v_sP - 0.5*v_salp;
v_5 = 0.3333*v_s0 - 0.3333*v_sP + 0.25*v_salp - sqrt(3)*0.25*v_sbet;
v_6 = 0.3333*v_s0 - 0.3333*v_sP + 0.25*v_salp + sqrt(3)*0.25*v_sbet;

W = [min([Vc_xy(1) + v_1 Vc_xy(4) + v_4]);
    min([Vc_xy(2) + v_2 Vc_xy(5) + v_5]);
    min([Vc_xy(3) + v_3 Vc_xy(6) + v_6]);
    -max([v_1 v_4]);
    -max([v_2 v_5]);
    -max([v_3 v_6])];

options = mpcActiveSetOptions;

% [Z, ~] = mpcActiveSetSolver(H,f,G_cc,W,Aeq,beq,false(size(W)),options);


% c_cc = -100*ones(2,1);
% b_cc = 100*ones(2,1);
% 
% [Z, ~] = BoxCQP_Nitmax(length(valbet_ref), H, f, c_cc, b_cc, x_uc , 100);
[Z, ~] = mpcActiveSetSolver(H,f,A_cc,b_cc,Aeq,beq,false(size(b_cc)),options);

W1 = [min([Vc_xy(1) + v_1 Vc_xy(4) + v_4]);
    min([Vc_xy(2) + v_2 Vc_xy(5) + v_5]);
    min([Vc_xy(3) + v_3 Vc_xy(6) + v_6]);
    max([v_1 v_4]);
    max([v_2 v_5]);
    max([v_3 v_6])];

% lb = -vmax*ones(2,1);
% ub = vmax*ones(2,1);
% options = optimoptions('quadprog');
% options.Algorithm = 'active-set';
% options.Display = 'off';
% Z = quadprog(H,f,[],[],[],[],lb,ub,v_opt,options);
% Y = Z';

valbet_delta = En*Z;
ialbet_delr = ialbet_deltar;
% valbet = valbet_delta;
deb = W1;
% v_opt = valbet_delta;

== matlab function M2C_IM_CL_V1_NCADMM_Sim/SM_MainCPU/Modo común ==
  settings: updateMethod=DISCRETE  sampleTime=ts
  data: in input; wb parameter; vo output; mag_ang output
function [vo, mag_ang] = fcn(in, wb)

% V_dc = in(1)/2;
V_dc = 500/2;
w_st = in(2);
t = in(3);
En = in(4);

wo = 1*150*2*pi;
k = 0.8;
% if abs(w) < 2*pi*11
%     k = 0.8;
% else
%     k = 0.8;
% end

k2 = 1;
% if abs(w) > 2*pi*15
%     k2 = 1.1;
% end
% 
% if abs(w) > 2*pi*20
%     k = 0.3*0;
% end


V_o = k*V_dc*(1 - k2*abs(w_st)/wb);

if V_o >= k*V_dc
    V_o = k*V_dc;
elseif V_o <= -k*V_dc
    V_o = -k*V_dc;
end

% if abs(w) < 2*pi*10
%     vo = V_o*sign(sin(wo*t));
% else
%     wo = 150*2*pi;
%     vo = V_o*sin(wo*t);
% end


% vo = V_o*sign(sin(wo*t));
vo = En*V_o*sin(wo*t);
mag_ang = En*[V_o ; wo*t];

== matlab function M2C_IM_CL_V1_NCADMM_Sim/SM_MainCPU/TEB Control Proportional Integral Control1 ==
  settings: updateMethod=DISCRETE  sampleTime=ts
  data: in input; i_dc output; prmt_TEB parameter; deb output
function [i_dc,deb] = fcn(in, prmt_TEB)
% 3 inputs
% 1 output
% 5 parameters



imax = prmt_TEB(3);
ts = prmt_TEB(7);
wn_teb = prmt_TEB(8);
dam = prmt_TEB(9);
e = prmt_TEB(10);


% Vsc_0 = in(1);
En_total = in(1);
Vdc_ref = in(2);
Pff = in(3);
Vdc = in(4);
En = in(5);


Vsc_0 = En_total;


K_teb = Vdc;

d0_teb = 1; 
n0_teb = ts*K_teb;

aux_teb = -dam*wn_teb*ts;
a1_teb = -2*e^(aux_teb)*cos(wn_teb*ts*sqrt(1-dam^2));
a2_teb = e^(-2*dam*wn_teb*ts);

Kct = (a1_teb + d0_teb + 1)/n0_teb;
nct = (d0_teb - a2_teb)/(a1_teb + d0_teb + 1);


% error
persistent a 
if isempty(a)
    a = 0;
end

% % antiwindup signal
persistent u
if isempty(u)
    u = 0;
end


%% PI antiwindup
e1 = (Vdc_ref - Vsc_0);

a = (nct - 1)*u/Kct + a*nct;
u = (e1 - a)*Kct;


if u >= imax
    u = imax;
elseif u <= -imax
    u = -imax;
end

deb = u;
i_dc = En*(u - 0*Pff/(Vdc));

== matlab function M2C_IM_CL_V1_NCADMM_Sim/SM_MainCPU/V_dc--->En_ref ==
  settings: updateMethod=DISCRETE  sampleTime=ts
  data: u input; y output; n parameter; C_sm parameter
function y = fcn(u, n, C_sm)

% u = 10*0 + u/n;
y = 6*0.5*C_sm*n*(u)^2;

== matlab function M2C_IM_CL_V1_NCADMM_Sim/SM_MainCPU/MATLAB Function1 ==
  data: u input; y output
function y = fcn(u)
U=[u(1:3)';u(4:6)'];
T=[1/2 1/2;1 -1];
C=[2/3 0 1/3;-1/3 1/sqrt(3) 1/3;-1/3 -1/sqrt(3) 1/3];
X=T*U*C;
y = [X(1,:)';X(2,:)'];

== matlab function M2C_IM_CL_V1_NCADMM_Sim/SM_MainCPU/LCB1/Greedy2 ==
  settings: updateMethod=DISCRETE  sampleTime=ts
  data: Vc_xy input; i_xy input; m_xy output; prmt_LCB parameter; Vcr_xy input; EN input; Op_all input; EN_TEB input
function m_xy  = fcn(Vc_xy, i_xy, prmt_LCB, Vcr_xy, EN, Op_all, EN_TEB)

%% Local Balance P controller
n = prmt_LCB(1) ; Vc_prom = prmt_LCB(2); Kc = prmt_LCB(3);

m_xyh = zeros(4,2);
% m_xyl = zeros(4,1);

Vc1 = Vc_xy(1) ; Vc2 = Vc_xy(2); Vc3 = Vc_xy(3); Vc4 = Vc_xy(4);

% d1 = (Vc_prom - Vc1);
% d2 = (Vc_prom - Vc2);
% d3 = (Vc_prom - Vc3);
% d4 = (Vc_prom - Vc4);

d = [Vc1 1; Vc2 2; Vc3 3; Vc4 4];
st_two_w = zeros(2,2);
st_two_l = zeros(2,2);

st_three = zeros(2,2);

% Stage 1 
if Vc1 > Vc2
    st_two_w(1,:) = d(1,:);
    st_two_l(1,:) = d(2,:);
else
    st_two_w(1,:) = d(2,:);
    st_two_l(1,:) = d(1,:);
end
if Vc3 > Vc4
    st_two_w(2,:) = d(3,:);
    st_two_l(2,:) = d(4,:);
else
    st_two_w(2,:) = d(4,:);
    st_two_l(2,:) = d(3,:);
end

% Stage 2
if st_two_w(1,1) > st_two_w(2,1)
    m_xyh(1,:) = st_two_w(1,:);
    st_three(1,:) = st_two_w(2,:);
else
    m_xyh(1,:) = st_two_w(2,:);
    st_three(1,:) = st_two_w(1,:);
end
if st_two_l(1,1) < st_two_l(2,1)
    m_xyh(4,:) = st_two_l(1,:);
    st_three(2,:) = st_two_l(2,:);
else
    m_xyh(4,:) = st_two_l(2,:);
    st_three(2,:) = st_two_l(1,:);
end

%Stage 3
if st_three(1,1) > st_three(2,1)
    m_xyh(2,:) = st_three(1,:);
    m_xyh(3,:) = st_three(2,:);
else
    m_xyh(2,:) = st_three(2,:);
    m_xyh(3,:) = st_three(1,:);
end

if sign(i_xy) > 0
    m_xyh = flip(m_xyh);
end

u_xy = m_xyh(:,1); % Orden de tensiones
n_xy = m_xyh(:,2); % Submodulo al que pertenecen

m_xy = zeros(4,1);
u_sigma = 0;

for i = 1:4
    l = n_xy(i);
    if u_sigma + u_xy(i) <= Vcr_xy
        m_xy(l) = 1;
        u_sigma = u_sigma + u_xy(i);
    else
        m_xy(l) = (Vcr_xy - u_sigma)/u_xy(i);
        if m_xy(l) < 0
            m_xy(l) = 0;
        end
%         if m_xy(l) > 1
%             m_xy(l) = 1;
%         end
        break
    end
end

% m_xy = EN*m_xy;


if Op_all == 1 && EN_TEB == 0
    m_xy = ones(4,1);
else
    m_xy = EN*m_xy;
end






% % Sort h
% for i = 1:4
%     for j = 1:4
%     if i ~= j
%         if d(i) > d(j)
%             m_xyh(i) = m_xyh(i) + 1;
%         end
%     end
%     end
% end
% 
% % Sort l
% for i = 1:4
%     for j = 1:4
%     if i ~= j
%         if d(i) < d(j)
%             m_xyl(i) = m_xyl(i) + 1;
%         end
%     end
%     end
% end
% 
% if sign(i_xy) >= 0
%     m_xy = m_xyh;
% else
%     m_xy = m_xyl;
% end



% for i = 1:4
%     m_xy(i) = Vcrp(i) + d(i);
% end

== matlab function M2C_IM_CL_V1_NCADMM_Sim/SM_MainCPU/Modo común1 ==
  settings: updateMethod=DISCRETE  sampleTime=ts
  data: in input; wb parameter; vo output; mag_ang output
function [vo, mag_ang] = fcn(in, wb)

% V_dc = in(1)/2;
V_dc = 500/2;
w_st = in(2);
t = in(3);
En = in(4);

wo = 1*200*2*pi;
k = 0.7;
% if abs(w) < 2*pi*11
%     k = 0.8;
% else
%     k = 0.8;
% end

k2 = 3;
% if abs(w) > 2*pi*15
%     k2 = 1.1;
% end
% 
% if abs(w) > 2*pi*20
%     k = 0.3*0;
% end


V_o = k2*k*V_dc;

% if V_o >= k2*k*V_dc
%     V_o = k2*k*V_dc;
% elseif V_o <= -k2*k*V_dc
%     V_o = -k2*k*V_dc;
% end

% if abs(w) < 2*pi*10
%     vo = V_o*sign(sin(wo*t));
% else
%     wo = 150*2*pi;
%     vo = V_o*sin(wo*t);
% end


% vo = V_o*sign(sin(wo*t));
vo = En*V_o*sin(wo*t);
if vo > k*V_dc*(1 - abs(w_st)/wb)
    vo = k*V_dc*(1 - abs(w_st)/wb);
elseif vo < -k*V_dc*(1 - abs(w_st)/wb)
    vo = -k*V_dc*(1 - abs(w_st)/wb);
end

if vo >= k*V_dc
    vo = k*V_dc;
elseif vo <= -k*V_dc
    vo = -k*V_dc;
end
mag_ang = En*[V_o ; wo*t];

== matlab function M2C_IM_CL_V1_NCADMM_Sim/SM_MainCPU/dq --> abc ==
  settings: updateMethod=DISCRETE  sampleTime=ts
  data: dq input; abc output; Theta_s input
function abc = fcn(dq, Theta_s)

Tab = [cos(Theta_s) -sin(Theta_s);
      cos(Theta_s-2*pi/3) -sin(Theta_s-2*pi/3);
      cos(Theta_s+2*pi/3) -sin(Theta_s+2*pi/3)];
abc = Tab*dq;

== matlab function M2C_IM_CL_V1_NCADMM_Sim/SM_MainCPU/Vc_kxy --> Vc_xy1 ==
  settings: updateMethod=DISCRETE  sampleTime=ts
  data: Vc_ap input; En_total output; Vc_bp input; Vc_cp input; Vc_an input; Vc_bn input; Vc_cn input; C_sm parameter
function En_total  = fcn(Vc_ap, Vc_bp, Vc_cp, Vc_an, Vc_bn, Vc_cn, C_sm)

Vc_xy_sq = zeros(6,1);


Vc_xy_sq(1) = Vc_ap(1)^2 + Vc_ap(2)^2 + Vc_ap(3)^2 + Vc_ap(4)^2;
Vc_xy_sq(2) = Vc_bp(1)^2 + Vc_bp(2)^2 + Vc_bp(3)^2 + Vc_bp(4)^2;
Vc_xy_sq(3) = Vc_cp(1)^2 + Vc_cp(2)^2 + Vc_cp(3)^2 + Vc_cp(4)^2;
Vc_xy_sq(4) = Vc_an(1)^2 + Vc_an(2)^2 + Vc_an(3)^2 + Vc_an(4)^2;
Vc_xy_sq(5) = Vc_bn(1)^2 + Vc_bn(2)^2 + Vc_bn(3)^2 + Vc_bn(4)^2;
Vc_xy_sq(6) = Vc_cn(1)^2 + Vc_cn(2)^2 + Vc_cn(3)^2 + Vc_cn(4)^2;

En_total = 0.5*C_sm*sum(Vc_xy_sq);

== matlab function M2C_IM_CL_V1_NCADMM_Sim/SM_MainCPU/Vc_kxy --> Vc_xy2 ==
  settings: updateMethod=DISCRETE  sampleTime=ts
  data: Vc_ap input; V_xy output; Vc_bp input; Vc_cp input; Vc_an input; Vc_bn input; Vc_cn input; d_ap input; d_bp input; d_cp input; d_an input; d_bn input; d_cn input
function V_xy  = fcn(Vc_ap,Vc_bp,Vc_cp,Vc_an,Vc_bn,Vc_cn,d_ap,d_bp,d_cp,d_an,d_bn,d_cn)

V_xy = zeros(6,1);

V_xy(1) = Vc_ap(1)*d_ap(1) + Vc_ap(2)*d_ap(2) + Vc_ap(3)*d_ap(3) + Vc_ap(4)*d_ap(4);
V_xy(2) = Vc_bp(1)*d_bp(1) + Vc_bp(2)*d_bp(2) + Vc_bp(3)*d_bp(3) + Vc_bp(4)*d_bp(4);
V_xy(3) = Vc_cp(1)*d_cp(1) + Vc_cp(2)*d_cp(2) + Vc_cp(3)*d_cp(3) + Vc_cp(4)*d_cp(4);
V_xy(4) = Vc_an(1)*d_an(1) + Vc_an(2)*d_an(2) + Vc_an(3)*d_an(3) + Vc_an(4)*d_an(4);
V_xy(5) = Vc_bn(1)*d_bn(1) + Vc_bn(2)*d_bn(2) + Vc_bn(3)*d_bn(3) + Vc_bn(4)*d_bn(4);
V_xy(6) = Vc_cn(1)*d_cn(1) + Vc_cn(2)*d_cn(2) + Vc_cn(3)*d_cn(3) + Vc_cn(4)*d_cn(4);
